simulink model "PartC"  (R2021b)
settings: Solver=VariableStepAuto  StartTime=0.0  StopTime=2/1000  RelTol=1e-3
libraries: commanapbnd3 x1
settings Model: Creator=Youssef Islam  LastModifiedBy=Youssef Islam

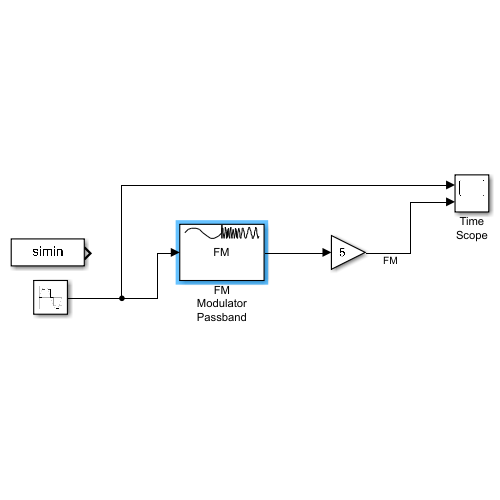
[thumbnail: Simulink's stored preview of the top-level diagram]
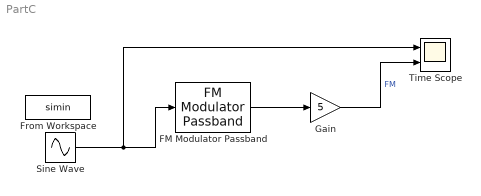
== system PartC ==
  FM Modulator Passband : commanapbnd3/FM Modulator Passband  Fc=20000  Ph=0  Kc=kf
      settings: SourceProductBaseCode=CM
  From Workspace : FromWorkspace  VariableName=simin  SampleTime=0.000001
  Gain : Gain  Gain=5
  Sine Wave : Sin  Amplitude=3  Frequency=2*pi*1000  SampleTime=0.00000001
  Time Scope : Scope  NumInputPorts=2
  wires:
  FM Modulator Passband/1 -> Gain/1
  Gain/1 -> Time Scope/2  "FM"
  Sine Wave/1 -> Time Scope/1, FM Modulator Passband/1
